simulink model "lab4pt2OFI"  (Simulink 8.0)
settings: Solver=ode1  StartTime=0.0  StopTime=10  FixedStep=0.002  RelTol=1e-3
libraries: simulink_extras x1
settings Model: Creator=vukovic8  LastModifiedBy=vukovic8  ExtModeTrigDuration=5000
settings SolverCC: PositivePriorityOrder=on
settings RTWCC: SystemTargetFile=quarc_win64.tlc  TemplateMakefile=quarc_default_tmf  Description=QUARC Win64 Target  ProcessScript=quarc_win64_make_rtw_hook
settings STFCustomTargetCC: TargetPreCompLibLocation=C:\PROGRA~3\QUARC\lib\2012b\win64\release  CodeReplacementLibrary=ANSI_C  GeneratePreprocessorConditionals=Disable all  CombineOutputUpdateFcns=on  GRTInterface=off  SystemTargetFile=quarc_win64.tlc
settings GRTTargetCC: TargetPreCompLibLocation=C:\PROGRA~3\QUARC\lib\2012b\win64\release  ParMdlRefBuildCompliant=off  CompOptLevelCompliant=off  ConcurrentExecutionCompliant=off  MatFileLogging=off  ExtMode=on  ExtModeMexFile=quarc_comm

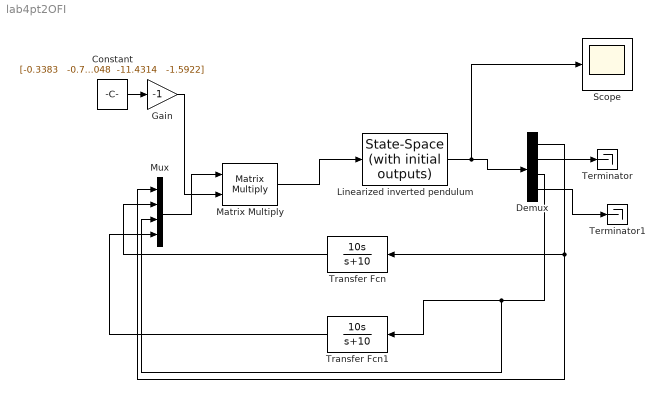
== system lab4pt2OFI ==
  Constant : Constant  Value="[-0.3383   -0.7048  -11.4314   -1.5922]"
  Demux : Demux
  Gain : Gain  Gain=-1
  Linearized inverted pendulum : simulink_extras/Additional Linear/State-Space (with initial outputs)  A=[0,1,0,0; 0,0,-4.5138,0; 0,0,0,1; 0,0,47.1744,0]  B=[0; 2.1978; 0; -7.2535]  C=eye(4)  D=[0;0;0;0]  U0=1  Y0=[0; 0; 0.035; 0.01]
  Matrix Multiply : Product  Multiplication=Matrix(*)
  Mux : Mux
  Scope : Scope
      settings: ShowLegends=on
  Terminator : Terminator
  Terminator1 : Terminator
  Transfer Fcn : TransferFcn  Numerator=[10 0]  Denominator=[1 10]
  Transfer Fcn1 : TransferFcn  Numerator=[10 0]  Denominator=[1 10]
  wires:
  Constant/1 -> Gain/1
  Linearized inverted pendulum/1 -> Scope/1, Demux/1
  Demux/2 -> Terminator/1
  Demux/4 -> Terminator1/1
  Demux/1 -> Mux/1, Transfer Fcn/1
  Demux/3 -> Mux/3, Transfer Fcn1/1
  Matrix Multiply/1 -> Linearized inverted pendulum/1
  Mux/1 -> Matrix Multiply/1
  Gain/1 -> Matrix Multiply/2
  Transfer Fcn/1 -> Mux/2
  Transfer Fcn1/1 -> Mux/4
